simulink model "ProyectoSC"  (R2025b)
settings: Solver=FixedStepAuto  StartTime=0.0  StopTime=Inf  RelTol=1e-3
model workspace (MAT data in the model file):
  alm1 : string (value not decoded)
libraries: slrealtimeiplib x3, sldrtlib x1
(part 2 of 2)

== stateflow chart ProyectoSC/Chart ==
  state Estadoinicial
    Home=1;
  state ModoManual
    state Mov
      during:
      sendmsg=0;
      TURNO=0;
    state EspJug
      during:
      sendmsg=0;
      MOD=4;
      TURNO=1;
    state Inicio
      MOD=1;
    state EspRiv
      during:
      sendmsg=0;
      MOD=4;
      TURNO=0;
    (default) -> ModoManual.Inicio
    ModoManual.Inicio -> EspJug [order 1] : [Init==0]{sendmsg=1}
    EspJug -> ModoManual.Mov : [DecJug==1]{sendmsg=1}
    ModoManual.Inicio -> ModoManual.EspRiv [order 2] : [Init==1]{sendmsg=1}
    ModoManual.EspRiv -> EspJug : [FTU==1]
    ModoManual.Mov -> ModoManual.EspRiv : [FTUJ==1]
  state ModoAutomatico
    state Mov
      during:
      sendmsg=0;
    state Inicio
      MOD=2;
    state EspOrd
      during:
      sendmsg=0;
      MOD=5;
    state EspRiv
      during:
      sendmsg=0;
      MOD=5;
    ModoAutomatico.Inicio -> EspOrd [order 1] : [Init==0]{sendmsg=1}
    EspOrd -> ModoAutomatico.Mov : [DecOrd==1]{sendmsg=1}
    (default) -> ModoAutomatico.Inicio
    ModoAutomatico.Inicio -> ModoAutomatico.EspRiv [order 2] : [Init==1]{sendmsg=1}
    ModoAutomatico.EspRiv -> EspOrd : [FTU==1]
    ModoAutomatico.Mov -> ModoAutomatico.EspRiv : [FTUJ==1]
  (default) -> Estadoinicial
  Estadoinicial -> ModoManual [order 1] : [Start==1 && Home==1 && Modo==1]
  ModoManual -> Estadoinicial : [FinPartida==1]
  ModoAutomatico -> Estadoinicial : [FinPartida==1]
  Estadoinicial -> ModoAutomatico [order 2] : [Start==1 && Home==1 && Modo==2]
  data: DecJug input; FinPartida input; FTU input; Init input; Modo input; Start input; DecOrd input size=1; sendmsg output; Home local; MOD output; FTUJ input; TURNO output

== matlab function ProyectoSC/T ==
  data: tablero input; c1 output; c2 output; c3 output; c4 output; c5 output; c6 output; c7 output; c8 output; c9 output
function [c1, c2, c3, c4, c5, c6, c7, c8, c9] = InterpretarTablero(tablero)
%#codegen
% Extrae 9 variables escalares del vector 1x9 del tablero.
%
% Entrada:
%   tablero: vector double 1x9 (0=vacío, 1=rival, 2=propio)
%
% Salidas:
%   c1-c9: valor de cada casilla
%
% Mapeo:  1 2 3
%         4 5 6
%         7 8 9

c1 = tablero(1); c2 = tablero(2); c3 = tablero(3);
c4 = tablero(4); c5 = tablero(5); c6 = tablero(6);
c7 = tablero(7); c8 = tablero(8); c9 = tablero(9);

end

== matlab function ProyectoSC/MATLAB Function1 ==
  data: turno input; mensaje output
function mensaje = MensajeTurno(turno)
%#codegen
% Devuelve un mensaje de estado segun el valor de entrada.
% Entrada:
%   turno: 0 o 1
% Salida:
%            0 -> 'Espera'
%            1 -> 'Te toca jugar'

if turno == 1
    mensaje = "Te toca jugar";
else
    mensaje = "Espera";
end

== matlab function ProyectoSC/Send ==
  data: data_out output; modo input; origen input; destino input
function data_out = SimulinkEmisor(modo, origen, destino)
% Formatea mensajes TCP/IP para enviar al robot Ned2.
% modo:    1=INI MAN | 2=INI AUT | 3=INI COM | 4=MOV (con origen/destino) | 5=MOV (solo) | 0=MOV (con origen/destino)
% origen:  1-9 (tablero) | 11-13 (alm1-alm3)
% destino: 1-9 (tablero)
%
% data_out es siempre uint8[1×32] de tamaño fijo.

% Buffer fijo de 32 bytes relleno con LF (char 10)
data_out = uint8(10 .* ones(1, 32, 'uint8'));

msg = char(zeros(1, 0));

modo_id = round(double(modo));
if modo_id >= 1 && modo_id <= 3
    % ── Mensaje INI ──────────────────────────────────────────
    if modo_id == 1
        msg = ['INI MAN' char(10)];
    elseif modo_id == 2
        msg = ['INI AUT' char(10)];
    else
        msg = ['INI COM' char(10)];
    end
else
    % ── Mensaje MOV ──────────────────────────────────────────
    if modo_id == 5
        % Modo 5: enviar solo "MOV" sin parámetros
        msg = ['MOV' char(10)];
    else
        % Modo 0, 4 o resto: enviar "MOV origen destino"
        orig_id = round(double(origen));
        dest_id = round(double(destino));

        orig_str = char(zeros(1, 0));
        if orig_id == 11
            orig_str = 'alm1';
        elseif orig_id == 12
            orig_str = 'alm2';
        elseif orig_id == 13
            orig_str = 'alm3';
        elseif orig_id >= 1 && orig_id <= 9
            orig_str = char(real(48 + orig_id));
        end

        if ~isempty(orig_str) && dest_id >= 1 && dest_id <= 9
            msg = ['MOV ' orig_str ' ' char(real(48 + dest_id)) char(10)];
        end
    end
end

% ── Copiar msg en data_out byte a byte (tamaño siempre 32) ───
if ~isempty(msg)
    b  = uint8(msg);
    nb = min(numel(b), 31);
    for k = 1:nb
        data_out(k) = b(k);
    end
    data_out(32) = uint8(10);
end
